simulink model "pmsm_discrete_model"  (R2023b)
settings: Solver=FixedStepDiscrete  StartTime=0.0  StopTime=0.05  FixedStep=Ts  RelTol=1e-3
model workspace (MATLAB code in the model file):
  | % Phase 3 — Discrete PMSM Model Parameters (Day-6 skeleton)
  | % Note: Values are placeholders for numerical closure only.
  | %       They do not represent final design commitments.
  | 
  | % --- Simulation / discretisation ---
  | Ts = 1e-6;              % [s] discrete step (aligned with Phase-3 switching env)
  | 
  | % --- PMSM electrical parameters (placeholder) ---
  | Rs = 0.38;              % [ohm] stator resistance
  | Ld = 1e-3;              % [H] d-axis inductance (placeholder)
  | Lq = 1e-3;              % [H] q-axis inductance (placeholder)
  | lambda_f = 0.1;         % [Wb] PM flux linkage (placeholder)
  | 
  | % --- Optional: governance note (kept as text, not used in equations) ---
  | pmsm_param_note = "Day-6 placeholders for model closure only; no calibration intended.";
settings Model: Creator=hwma  LastModifiedBy=hwma

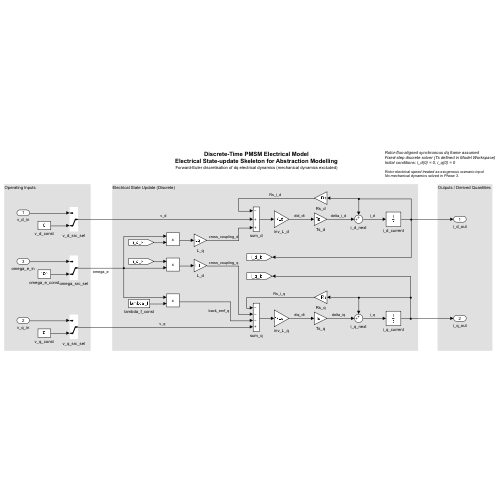
[thumbnail: Simulink's stored preview of the top-level diagram]
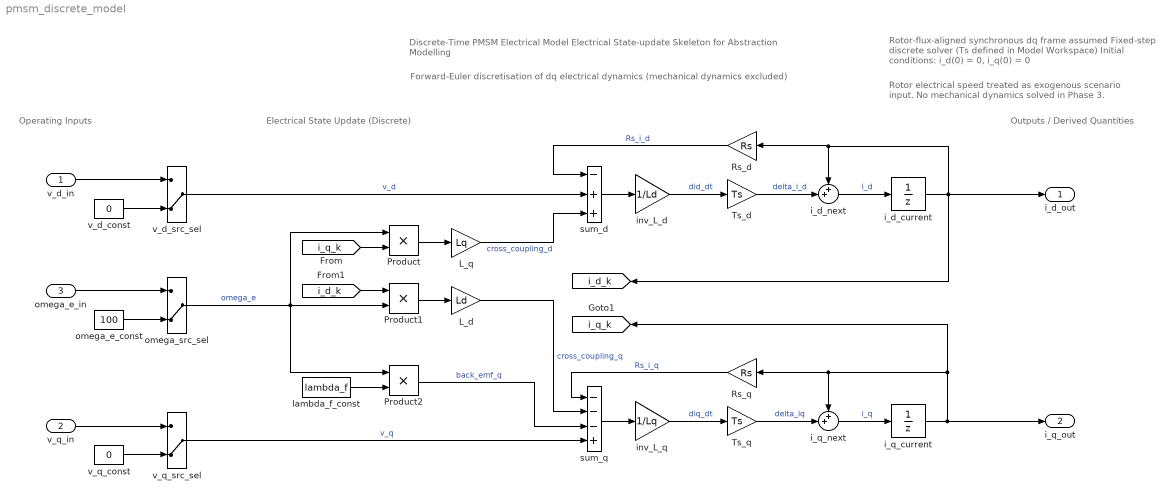
== system pmsm_discrete_model ==
  note: Rotor-flux-aligned synchronous dq frame assumed
      | Fixed-step discrete solver (Ts defined in Model Workspace)
      | Initial conditions: i_d(0) = 0, i_q(0) = 0
  note: Operating Inputs
  note: Rotor electrical speed treated as exogenous scenario input.
      | No mechanical dynamics solved in Phase 3.
  note: Forward-Euler discretisation of dq electrical dynamics (mechanical dynamics excluded)
  note: Discrete-Time PMSM Electrical Model
      | Electrical State-update Skeleton for Abstraction Modelling
  note: Electrical State Update (Discrete)
  note: Outputs / Derived Quantities
  v_d_in : Inport
  v_q_in : Inport  Port=2
  omega_e_in : Inport  Port=3
  L_d : Gain  Gain=Ld
  L_q : Gain  Gain=Lq
  Product : Product
  Product1 : Product
  Product2 : Product
  Rs_d : Gain  Gain=Rs
  Rs_q : Gain  Gain=Rs
  Ts_d : Gain  Gain=Ts
  Ts_q : Gain  Gain=Ts
  i_d_current : UnitDelay  SampleTime=Ts  HasFrameUpgradeWarning=on
  i_d_next : Sum  Inputs=++|
  i_q_current : UnitDelay  SampleTime=Ts  HasFrameUpgradeWarning=on
  i_q_next : Sum  Inputs=++|
  inv_L_d : Gain  Gain=1/Ld
  inv_L_q : Gain  Gain=1/Lq
  lambda_f_const : Constant  Value=lambda_f
  omega_e_const : Constant  Value=100
  omega_src_sel : ManualSwitch  CurrentSetting=0
  sum_d : Sum  Inputs=-++
  sum_q : Sum  Inputs=---+
  v_d_const : Constant  Value=0
  v_d_src_sel : ManualSwitch  CurrentSetting=0
  v_q_const : Constant  Value=0
  v_q_src_sel : ManualSwitch  CurrentSetting=0
  i_d_out : Outport
  i_q_out : Outport  Port=2
  tag scope: i_d_k=global, i_q_k=global
  wires:
  v_d_in/1 -> v_d_src_sel/1
  v_d_const/1 -> v_d_src_sel/2
  v_q_const/1 -> v_q_src_sel/2
  v_q_in/1 -> v_q_src_sel/1
  omega_e_in/1 -> omega_src_sel/1
  omega_e_const/1 -> omega_src_sel/2
  v_d_src_sel/1 -> sum_d/2  "v_d"
  v_q_src_sel/1 -> sum_q/4  "v_q"
  i_d_current/1 -> [i_d_k], i_d_out/1, Rs_d/1, i_d_next/1
  Rs_d/1 -> sum_d/1  "Rs_i_d"
  Product/1 -> L_q/1
  L_q/1 -> sum_d/3  "cross_coupling_d"
  sum_d/1 -> inv_L_d/1
  inv_L_d/1 -> Ts_d/1  "did_dt"
  i_d_next/1 -> i_d_current/1  "i_d"
  inv_L_q/1 -> Ts_q/1  "diq_dt"
  i_q_current/1 -> i_q_out/1, [i_q_k], Rs_q/1, i_q_next/1
  L_d/1 -> sum_q/2  "cross_coupling_q"
  Product1/1 -> L_d/1
  omega_src_sel/1 -> Product2/1, Product1/2, Product/1  "omega_e"
  sum_q/1 -> inv_L_q/1
  Rs_q/1 -> sum_q/1  "Rs_i_q"
  Ts_d/1 -> i_d_next/2  "delta_i_d"
  Ts_q/1 -> i_q_next/2  "delta_iq"
  i_q_next/1 -> i_q_current/1  "i_q"
  lambda_f_const/1 -> Product2/2
  Product2/1 -> sum_q/3  "back_emf_q"
  [i_q_k] -> Product/2
  [i_d_k] -> Product1/1
